simulink model "simulinknurik"  (R2019a)
settings: Solver=VariableStepAuto  StartTime=0.0  StopTime=2  RelTol=1e-3
libraries: roblocks x3
settings Model: Creator=Нурлан  LastModifiedBy=Нурлан

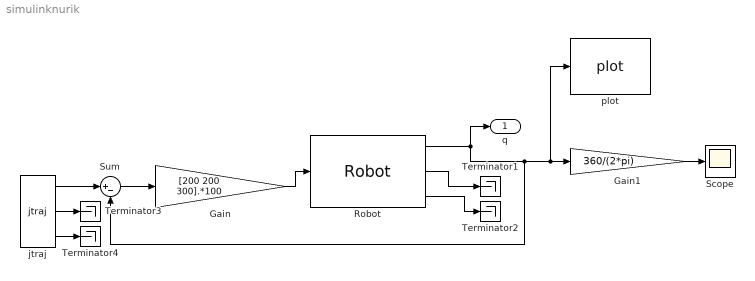
== system simulinknurik ==
  Gain : Gain  Gain=[200 200 300].*100
  Gain1 : Gain  Gain=360/(2*pi)
  Robot : roblocks/Arm/Robot  robot=robonurik.nofriction  q0=[0 0 0]
  Scope : Scope
  Sum : Sum  Inputs=|+-
  Terminator{1..4} (4 alike) : Terminator
  jtraj : roblocks/Toolbox/jtraj  q0=[0 0 0]  qf=[pi/2 -pi/4 -pi/4]  tmax=2  ts=0.02
  plot : roblocks/Arm/plot  robot=robonurik  fps=25  holdplot=on
  q : Outport
  wires:
  Robot/1 -> q/1, Gain1/1, plot/1, Sum/2
  Robot/2 -> Terminator1/1
  Robot/3 -> Terminator2/1
  Sum/1 -> Gain/1
  jtraj/1 -> Sum/1
  Gain/1 -> Robot/1
  Gain1/1 -> Scope/1
  jtraj/3 -> Terminator4/1
  jtraj/2 -> Terminator3/1
